simulink model "ta6_nogravity"  (R2017a)
settings: Solver=VariableStepAuto  StartTime=0.0  StopTime=10.0  RelTol=1e-3
libraries: roblocks x2
settings Model: Creator=Administrator  LastModifiedBy=Administrator

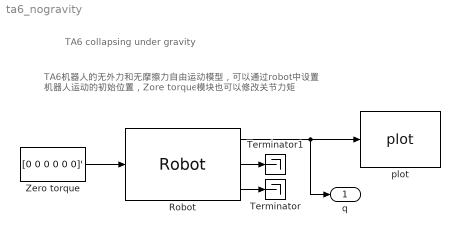
== system ta6_nogravity ==
  note: TA6机器人的无外力和无摩擦力自由运动模型，可以通过robot中设置
      | 机器人运动的初始位置，Zore torque模块也可以修改关节力矩
  note: TA6 collapsing under gravity
  Robot : roblocks/Arm/Robot  robot=ta6.nofriction  q0=[0 pi/2 pi/2 0 0 0]
  Terminator : Terminator
  Terminator1 : Terminator
  Zero torque : Constant  Value=[0 0 0 0 0 0]'
  plot : roblocks/Arm/plot  robot=ta6  fps=25  holdplot=on
  q : Outport
  wires:
  Robot/1 -> plot/1, q/1
  Robot/2 -> Terminator1/1
  Robot/3 -> Terminator/1
  Zero torque/1 -> Robot/1
